simulink model "detectGreenBallModel_test_start"  (R2018a)
settings: Solver=VariableStepAuto  StartTime=0.0  StopTime=Inf  RelTol=1e-3
undefined symbols (not defined in the file or in its folder): none, videoinput
libraries: simulink x1, imaqlib x1, visionsinks x1, visiontextngfix x1
settings Model: Creator=sseshadr  LastModifiedBy=scastro

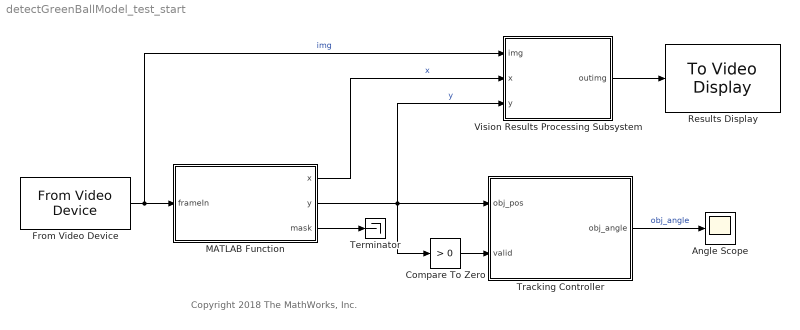
== system detectGreenBallModel_test_start ==
  note: Copyright 2018 The MathWorks, Inc.
  Angle Scope : Scope
  Compare To Zero : simulink/Logic and Bit Operations/Compare To Zero  relop=>  OutDataTypeStr=boolean  ZeroCross=off
  From Video Device : imaqlib/From Video Device  DeviceMenu=(none)  Device=winvideo 1 (Integrated Camera)  ObjConstructor=videoinput('winvideo', 1)  VideoFormatMenu=(none)  VideoFormat=RGB24_320x240  VideoSource=input1  ROIPosition=[0 0 240 320]  EnableHWTrigger=off  TriggerConfiguration=none/none  SampleTime=0.05  OutputPortsMode=One multidimensional signal  DataType=uint8  CanDoHWTrigger=no  ReturnedColorSpace=rgb  BlockHandle=1074.0005  ROIWidth=320  ROIHeight=240  ROIColumn=0  ROIRow=0  EngXMLPath=C:\Program Files\MATLAB\R2018a\toolbox\imaq\imaq\private  DevXMLPath=C:\ProgramData\MATLAB\SupportPackages\R2018a\toolbox\imaq\supportpackages\genericvideo\adaptor\win64  EngLibPath=C:\Program Files\MATLAB\R2018a\toolbox\imaq\imaqblks\imaqmex\win64  ColorSpace=rgb  BayerSensorAlignment=grbg
      settings: SourceProductName=Image Acquisition Toolbox
  MATLAB Function : MATLAB Function  TreatAsAtomicUnit=on
  Results Display : visionsinks/To Video Display  windowSizeMode=Normal  openAtMdlStart=on  fullScreen=off  videoWindowX=536805376  videoWindowY=536805376  saveWindowSize=off  videoWindowWidth=640  videoWindowHeight=480  inputColorFormat=RGB  inputType=Obsolete  imagePorts=One multidimensional signal  OutputDevice=On-screen video monitor  dataOrg=Column-major  isWindowOpen=off
      settings: SourceProductName=Computer Vision System Toolbox
  Terminator : Terminator
  Tracking Controller : Stateflow chart  TreatAsAtomicUnit=on
  Vision Results Processing Subsystem : Subsystem
  wires:
  Vision Results Processing Subsystem/1(outimg) -> Results Display/1
  MATLAB Function/1(x) -> Vision Results Processing Subsystem/2(x)  "x"
  MATLAB Function/3(mask) -> Terminator/1
  Compare To Zero/1 -> Tracking Controller/2(valid)
  From Video Device/1 -> MATLAB Function/1(frameIn), Vision Results Processing Subsystem/1(img)  "img"
  MATLAB Function/2(y) -> Tracking Controller/1(obj_pos), Vision Results Processing Subsystem/3(y), Compare To Zero/1  "y"
  Tracking Controller/1(obj_angle) -> Angle Scope/1  "obj_angle"

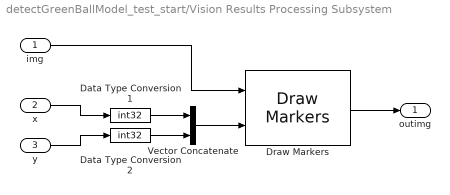
== system detectGreenBallModel_test_start/Vision Results Processing Subsystem ==
  img : Inport
  x : Inport  Port=2
  y : Inport  Port=3
  Data Type Conversion1 : DataTypeConversion  OutDataTypeStr=int32
  Data Type Conversion2 : DataTypeConversion  OutDataTypeStr=int32
  Draw Markers : visiontextngfix/Draw Markers  shape=Circle  size=3  fill=off  fillClrSource=Specify via dialog  display=Black  intensity=200  color=[200 255 100]  opacity=0.6  viewport=Entire image  antialiasing=off  inType=Obsolete  imagePorts=One multidimensional signal  prodOutputMode=Binary point scaling  prodOutputWordLength=32  prodOutputFracLength=14  memoryMode=Specify word length  memoryWordLength=16  memoryFracLength=15  roundingMode=Floor  overflowMode=off
      settings: SourceProductName=Computer Vision System Toolbox  SourceProductBaseCode=VP
  Vector Concatenate : Concatenate
  outimg : Outport
  wires:
  img/1 -> Draw Markers/1
  Vector Concatenate/1 -> Draw Markers/2
  Data Type Conversion2/1 -> Vector Concatenate/2
  Draw Markers/1 -> outimg/1
  Data Type Conversion1/1 -> Vector Concatenate/1
  y/1 -> Data Type Conversion2/1
  x/1 -> Data Type Conversion1/1

== stateflow chart detectGreenBallModel_test_start/Tracking Controller ==
  settings: sampleTime=1/15
  state dir = setDir(position) [function]
    (default) -> (junction 70)
    (junction 70) -> (junction 74) [order 1] : [position > 160]
    (junction 70) -> (junction 76) [order 2] : {dir = -1;}
    (junction 74) -> (junction 78) : {dir = 1;}
    (junction 78) -> (junction 76)
    (junction 76) -> (junction 86)
  state Tracking
    entry, during:
    obj_angle = objAngle(obj_pos);
    direction = setDir(obj_pos);
  state Waiting
    entry:
    i = 0;
    during:
    i = i + 1;
  state Seeking
    Seeking -> (junction 33) [order 1]
    (junction 33) -> (junction 40) [order 2]
    (junction 33) -> (junction 37) [order 1] : [direction==1]
    (junction 37) -> (junction 43) [order 2] : {direction=-1;}
    (junction 40) -> (junction 47) [order 2] : {direction=1;}
    (junction 37) -> (junction 43) [order 1] : [obj_angle < MAX_ANGLE]
        | {obj_angle = obj_angle + 10;}
    (junction 40) -> (junction 47) [order 1] : [obj_angle>-MAX_ANGLE]
        | {obj_angle = obj_angle - 10;}
    (junction 47) -> (junction 61)
    (junction 43) -> (junction 61)
  (default) -> Tracking
  Tracking -> Waiting : [~valid]
  Waiting -> Tracking [order 2] : [valid]
  Waiting -> Seeking [order 1] : [i>10]
  Seeking -> Tracking [order 1] : [valid]
  data: position function_input double; dir function_output double; pos function_input double; a function_output double; obj_pos input double; MAX_ANGLE local double =90; valid input; i local double; obj_angle output double; direction local double
  function a = objAngle(pos):
    | function a = objAngle(pos)
    | 
    | % a = atand((pos-200)/5000);
    | deadZone = 0.2;
    | 
    | a =(pos - 160)/160;
    | 
    | if abs(a)<(deadZone/2)
    |    a=0;
    | end
    | 
    | 
    | end

== matlab function detectGreenBallModel_test_start/MATLAB Function ==
  data: x output; frameIn input uint8 size=[240 320 3]; y output; mask output size=[240 320]
function [x,y,mask] = detectGreenBall(frameIn)
%#Codegen 

% This function thresholds the image based on threshold values submitted by
% the user

%% Setup the detector and initialize variables
persistent detector 
if isempty(detector)
    detector = vision.BlobAnalysis('BoundingBoxOutputPort',false,...
        'AreaOutputPort',false,'MinimumBlobArea',300, ...
        'MajorAxisLengthOutputPort',true,'MaximumCount', 10);
end
x = 0;
y = 0;
threshold = [107.00 225.00; 85.000 120.000; 82.000 121.000];

%% Threshold the image
frameIn = rgb2ycbcr(frameIn);
mask = (frameIn (:,:,1) >= threshold(1,1))& (frameIn (:,:,1) <= threshold(1,2))&...
    (frameIn (:,:,2) >= threshold(2,1))& (frameIn (:,:,2) <= threshold(2,2))&...
    (frameIn (:,:,3) >= threshold(3,1))& (frameIn (:,:,3) <= threshold(3,2));

[centroid,majorAxis] = detector(mask);


if ~isempty(majorAxis)
% Identify Largest Blob
    [~,mIdx] = max(majorAxis);
    C = centroid(mIdx,:);
    x = double(C(1));
    y = double(C(2));

end 

end
